simulink model "HeatExchanger"  (Simulink 8.3)
settings: Solver=ode4  StartTime=0.0  StopTime=10  FixedStep=delta_t  RelTol=1e-3
values from neighbouring files (symbols this model uses):
  delta_t = 1 / sensor_sampling_rate    (= 0.001)    [HeatExchanger_ps.m]    (also in steady_data_76rssi_30_1.mat = 0.1; steady_data_76rssi_40.mat = 0.1; steady_data_76rssi_iter.mat = 0.1; steady_data_76rssi_iter_reduce.mat = 0.1)
libraries: powerlib_meascontrol x3, simulink x1
settings Model: Creator=Rhine  LastModifiedBy=wangwenchen
settings OptimizationCC: ExpressionDepthLimit=2147483647
settings DebuggingCC: FcnCallInpInsideContextMsg=UseLocalSettings

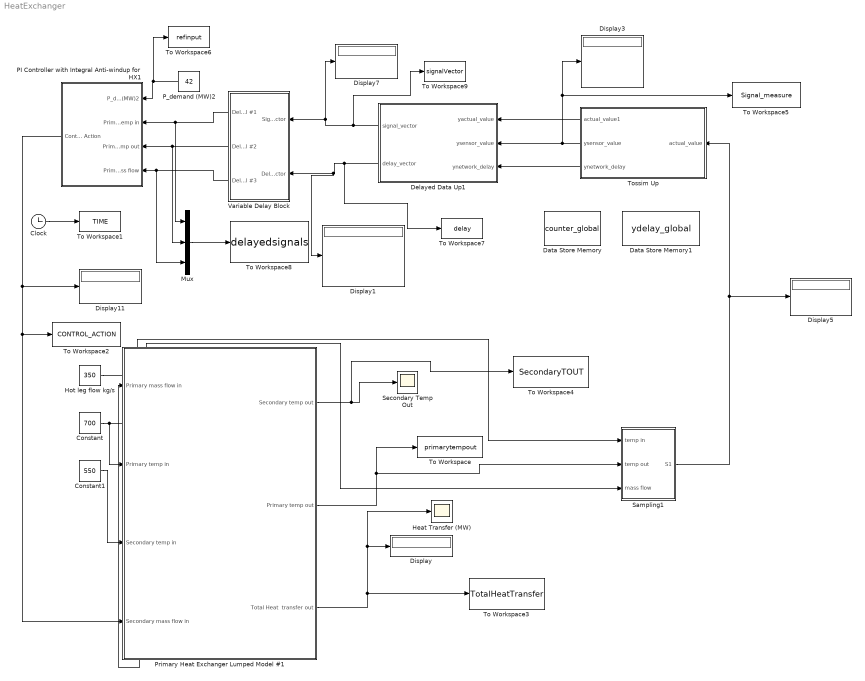
== system HeatExchanger ==
  Clock : Clock
  Constant : Constant  Value=700
  Constant1 : Constant  Value=550
  Data Store Memory : DataStoreMemory  DataStoreName=counter_global  ReadBeforeWriteMsg=warning  WriteAfterWriteMsg=warning  WriteAfterReadMsg=warning  OutDataTypeStr=int32
  Data Store Memory1 : DataStoreMemory  DataStoreName=ydelay_global  ReadBeforeWriteMsg=warning  WriteAfterWriteMsg=warning  WriteAfterReadMsg=warning  InitialValue=ones(10,1)  OutDataTypeStr=int32
  Delayed Data Up1 : MATLAB Function  TreatAsAtomicUnit=on  SystemSampleTime=0.1
  Display{,1,3,5,7,11} (6 alike) : Display
  Heat Transfer (MW) : Scope
      settings: TimeRange=30  YMin=23.3769  YMax=25.8377  SaveName=ScopeData3
  Hot leg flow kg/s : Constant  Value=350
  Mux : Mux  Inputs=3
  PI Controller with Integral Anti-windup for HX1 : Subsystem
  P_demand (MW)2 : Constant  Value=42
  Primary Heat Exchanger Lumped Model #1 : Subsystem
  Sampling1 : Subsystem
  Secondary Temp Out : Scope
      settings: YMin=639  YMax=640.4
  To Workspace : ToWorkspace  VariableName=primarytempout  SaveFormat=Timeseries  SampleTime=-1
  To Workspace1 : ToWorkspace  VariableName=TIME  SampleTime=-1
  To Workspace2 : ToWorkspace  VariableName=CONTROL_ACTION  SaveFormat=Timeseries  SampleTime=-1
  To Workspace3 : ToWorkspace  VariableName=TotalHeatTransfer  SaveFormat=Timeseries  SampleTime=-1
  To Workspace4 : ToWorkspace  VariableName=SecondaryTOUT  SaveFormat=Timeseries  SampleTime=-1
  To Workspace5 : ToWorkspace  VariableName=Signal_measure  SampleTime=-1
  To Workspace6 : ToWorkspace  VariableName=refinput  SaveFormat=Timeseries  SampleTime=-1
  To Workspace7 : ToWorkspace  VariableName=delay  SaveFormat=Timeseries  SampleTime=-1
  To Workspace8 : ToWorkspace  VariableName=delayedsignals  SaveFormat=Timeseries  SampleTime=-1
  To Workspace9 : ToWorkspace  VariableName=signalVector  SaveFormat=Timeseries  SampleTime=-1
  Tossim Up : MATLAB Function  TreatAsAtomicUnit=on  SystemSampleTime=0.1
  Variable Delay Block : Subsystem
  wires:
  Clock/1 -> To Workspace1/1
  Tossim Up/1(actual_value1) -> Delayed Data Up1/1(yactual_value)
  Sampling1/1(S1) -> Tossim Up/1(actual_value), Display5/1
  P_demand (MW)2/1 -> To Workspace6/1, PI Controller with Integral Anti-windup for HX1/1(P_demand (MW)2)
  Hot leg flow kg/s/1 -> Sampling1/3(mass flow), Primary Heat Exchanger Lumped Model #1/1(Primary mass flow in)
  Constant/1 -> Sampling1/1(temp in), Primary Heat Exchanger Lumped Model #1/2(Primary temp in)
  Constant1/1 -> Primary Heat Exchanger Lumped Model #1/3(Secondary temp in)
  Primary Heat Exchanger Lumped Model #1/2(Primary temp out) -> To Workspace/1, Sampling1/2(temp out)
  Primary Heat Exchanger Lumped Model #1/1(Secondary temp out) -> To Workspace4/1, Secondary Temp Out/1
  Variable Delay Block/1(Delayed signal #1) -> Mux/1, PI Controller with Integral Anti-windup for HX1/2(Primary temp in)
  Variable Delay Block/2(Delayed signal #2) -> PI Controller with Integral Anti-windup for HX1/3(Primary temp out), Mux/2
  Variable Delay Block/3(Delayed signal #3) -> Mux/3, PI Controller with Integral Anti-windup for HX1/4(Primary mass flow)
  PI Controller with Integral Anti-windup for HX1/1(Control Action) -> Display11/1, Primary Heat Exchanger Lumped Model #1/4(Secondary mass flow in), To Workspace2/1
  Primary Heat Exchanger Lumped Model #1/3("Total Heat  transfer out ") -> Heat Transfer (MW)/1, Display/1, To Workspace3/1
  Delayed Data Up1/1(signal_vector) -> To Workspace9/1, Display7/1, Variable Delay Block/1(Signal vector)
  Tossim Up/2(ysensor_value) -> Display3/1, To Workspace5/1, Delayed Data Up1/2(ysensor_value)
  Tossim Up/3(ynetwork_delay) -> Delayed Data Up1/3(ynetwork_delay)
  Delayed Data Up1/2(delay_vector) -> To Workspace7/1, Display1/1, Variable Delay Block/2(Delay vector)
  Mux/1 -> To Workspace8/1

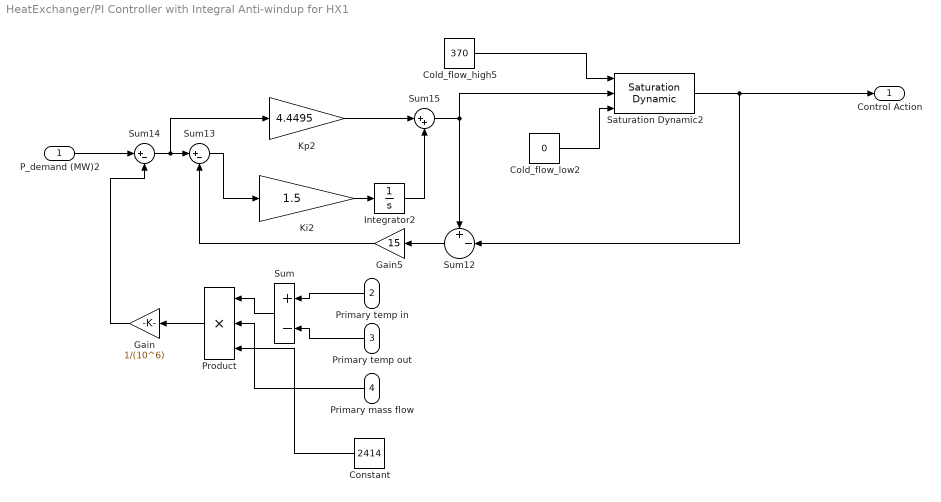
== system HeatExchanger/PI Controller with Integral Anti-windup for HX1 ==
  P_demand (MW)2 : Inport
  Primary temp in : Inport  Port=2
  Primary temp out : Inport  Port=3
  Primary mass flow : Inport  Port=4
  Cold_flow_high5 : Constant  Value=370
  Cold_flow_low2 : Constant  Value=0
  Constant : Constant  Value=2414
  Gain : Gain  Gain=1/(10^6)
  Gain5 : Gain  Gain=15
  Integrator2 : Integrator  InitialCondition=250
  Ki2 : Gain  Gain=1.5
  Kp2 : Gain  Gain=4.4495
  Product : Product  Inputs=3
  Saturation Dynamic2 : simulink/Discontinuities/Saturation Dynamic  OutMin=[]  OutMax=[]  OutDataTypeStr=Inherit: Same as second input  OutDataType=fixdt(1, 16)  OutScaling=2^-10  DoSatur=off
  Sum : Sum  Inputs=+-
  Sum12 : Sum  Inputs=+-|
  Sum13 : Sum  Inputs=|+-
  Sum14 : Sum  Inputs=|+-
  Sum15 : Sum  Inputs=|++
  Control Action : Outport
  wires:
  Product/1 -> Gain/1
  Cold_flow_low2/1 -> Saturation Dynamic2/3
  Cold_flow_high5/1 -> Saturation Dynamic2/1
  Sum14/1 -> Kp2/1, Sum13/1
  P_demand (MW)2/1 -> Sum14/1
  Sum12/1 -> Gain5/1
  Integrator2/1 -> Sum15/2
  Gain5/1 -> Sum13/2
  Sum13/1 -> Ki2/1
  Ki2/1 -> Integrator2/1
  Kp2/1 -> Sum15/1
  Saturation Dynamic2/1 -> Control Action/1, Sum12/2
  Sum15/1 -> Sum12/1, Saturation Dynamic2/2
  Primary temp in/1 -> Sum/1
  Primary temp out/1 -> Sum/2
  Sum/1 -> Product/1
  Primary mass flow/1 -> Product/2
  Constant/1 -> Product/3
  Gain/1 -> Sum14/2

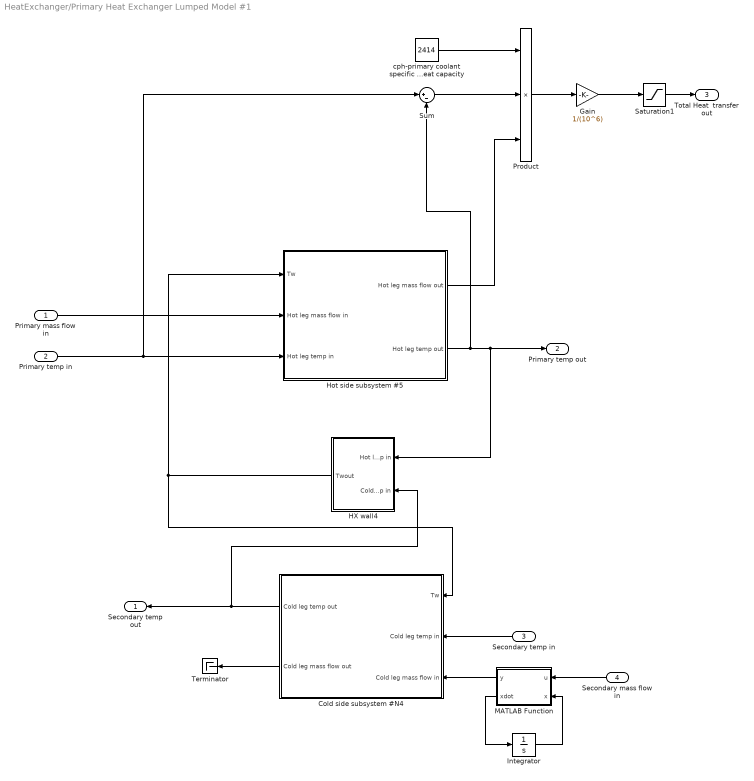
== system HeatExchanger/Primary Heat Exchanger Lumped Model #1 ==
  Primary mass flow in : Inport
  Primary temp in : Inport  Port=2
  Secondary temp in : Inport  Port=3
  Secondary mass flow in : Inport  Port=4
  Cold side subsystem #N4 : Subsystem
  Gain : Gain  Gain=1/(10^6)
  HX wall4 : Subsystem
  Hot side subsystem #5 : Subsystem
  Integrator : Integrator  InitialCondition=250
  MATLAB Function : MATLAB Function  TreatAsAtomicUnit=on
  Product : Product  Inputs=3
  Saturation1 : Saturate  UpperLimit=inf  LowerLimit=0
  Sum : Sum  Inputs=|+-
  Terminator : Terminator
  cph-primary coolant specific heat capacity : Constant  Value=2414
  Secondary temp out : Outport
  Primary temp out : Outport  Port=2
  "Total Heat  transfer out " : Outport  Port=3
  wires:
  Cold side subsystem #N4/1(Cold leg temp out) -> Secondary temp out/1, HX wall4/2(Cold leg temp in)
  Cold side subsystem #N4/2(Cold leg mass flow out) -> Terminator/1
  Primary mass flow in/1 -> Hot side subsystem #5/2(Hot leg mass flow in)
  Primary temp in/1 -> Hot side subsystem #5/3(Hot leg temp in), Sum/1
  Secondary mass flow in/1 -> MATLAB Function/1(u)
  Secondary temp in/1 -> Cold side subsystem #N4/2(Cold leg temp in)
  HX wall4/1(Twout) -> Cold side subsystem #N4/1(Tw), Hot side subsystem #5/1(Tw)
  Hot side subsystem #5/1(Hot leg mass flow out) -> Product/3
  Hot side subsystem #5/2(Hot leg temp out) -> HX wall4/1(Hot leg temp in), Primary temp out/1, Sum/2
  cph-primary coolant specific heat capacity/1 -> Product/1
  Sum/1 -> Product/2
  Product/1 -> Gain/1
  Gain/1 -> Saturation1/1
  MATLAB Function/1(y) -> Cold side subsystem #N4/3(Cold leg mass flow in)
  Saturation1/1 -> "Total Heat  transfer out "/1
  MATLAB Function/2(xdot) -> Integrator/1
  Integrator/1 -> MATLAB Function/2(x)

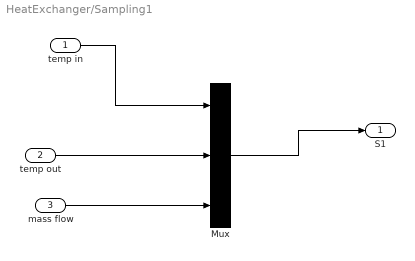
== system HeatExchanger/Sampling1 ==
  temp in : Inport
  temp out : Inport  Port=2
  mass flow : Inport  Port=3
  Mux : Mux  Inputs=3
  S1 : Outport
  wires:
  temp in/1 -> Mux/1
  temp out/1 -> Mux/2
  mass flow/1 -> Mux/3
  Mux/1 -> S1/1

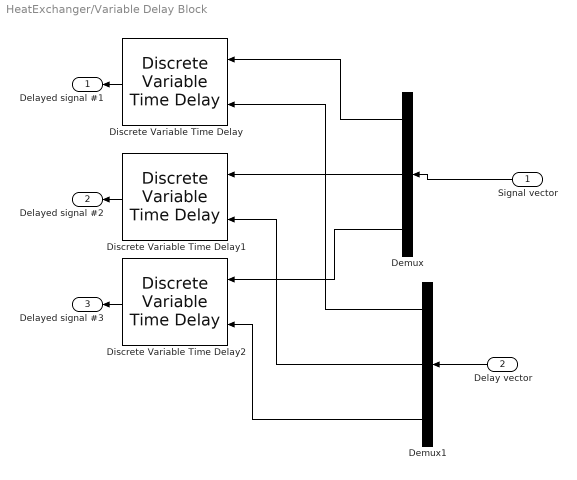
== system HeatExchanger/Variable Delay Block ==
  Signal vector : Inport
  Delay vector : Inport  Port=2
  Demux : Demux  Outputs=3
  Demux1 : Demux  Outputs=3
  Discrete Variable Time Delay : powerlib_meascontrol/Additional Components/Discrete Variable Time Delay  MaxDelay=2  InitialValue=700  Ts=delta_t  DFT=on
  Discrete Variable Time Delay1 : powerlib_meascontrol/Additional Components/Discrete Variable Time Delay  MaxDelay=2  InitialValue=650.29  Ts=delta_t  DFT=on
  Discrete Variable Time Delay2 : powerlib_meascontrol/Additional Components/Discrete Variable Time Delay  MaxDelay=2  InitialValue=350  Ts=delta_t  DFT=on
  Delayed signal #1 : Outport
  Delayed signal #2 : Outport  Port=2
  Delayed signal #3 : Outport  Port=3
  wires:
  Discrete Variable Time Delay1/1 -> Delayed signal #2/1
  Demux1/3 -> Discrete Variable Time Delay2/2
  Demux1/2 -> Discrete Variable Time Delay1/2
  Discrete Variable Time Delay2/1 -> Delayed signal #3/1
  Demux/3 -> Discrete Variable Time Delay2/1
  Demux/1 -> Discrete Variable Time Delay/1
  Demux1/1 -> Discrete Variable Time Delay/2
  Discrete Variable Time Delay/1 -> Delayed signal #1/1
  Signal vector/1 -> Demux/1
  Demux/2 -> Discrete Variable Time Delay1/1
  Delay vector/1 -> Demux1/1

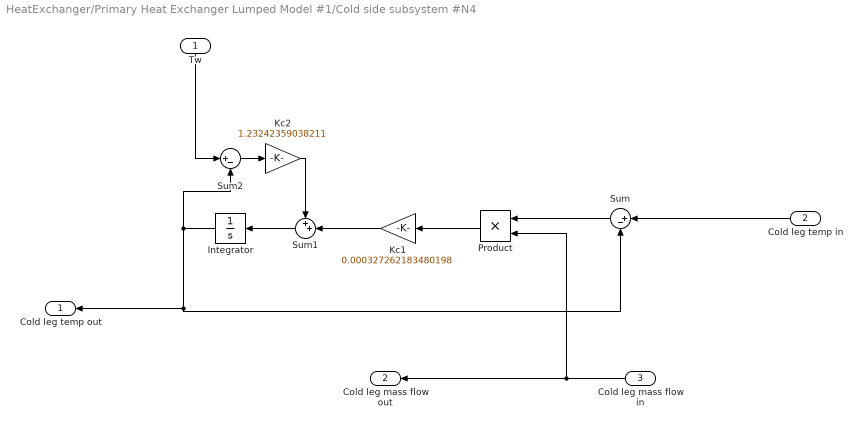
== system HeatExchanger/Primary Heat Exchanger Lumped Model #1/Cold side subsystem #N4 ==
  Tw : Inport
  Cold leg temp in : Inport  Port=2
  Cold leg mass flow in : Inport  Port=3
  Integrator : Integrator  InitialCondition=638.4
  Kc1 : Gain  Gain=0.000327262183480198
  Kc2 : Gain  Gain=1.23242359038211
  Product : Product
  Sum : Sum  Inputs=|+-
  Sum1 : Sum  Inputs=++|
  Sum2 : Sum  Inputs=|+-
  Cold leg temp out : Outport
  Cold leg mass flow out : Outport  Port=2
  wires:
  Cold leg temp in/1 -> Sum/1
  Integrator/1 -> Sum/2, Cold leg temp out/1, Sum2/2
  Sum2/1 -> Kc2/1
  Sum/1 -> Product/1
  Kc2/1 -> Sum1/1
  Sum1/1 -> Integrator/1
  Cold leg mass flow in/1 -> Cold leg mass flow out/1, Product/2
  Product/1 -> Kc1/1
  Kc1/1 -> Sum1/2
  Tw/1 -> Sum2/1

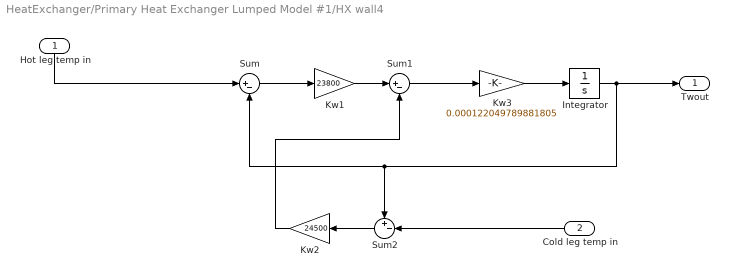
== system HeatExchanger/Primary Heat Exchanger Lumped Model #1/HX wall4 ==
  Hot leg temp in : Inport
  Cold leg temp in : Inport  Port=2
  Integrator : Integrator  InitialCondition=644.3
  Kw1 : Gain  Gain=23800
  Kw2 : Gain  Gain=24500
  Kw3 : Gain  Gain=0.000122049789881805
  Sum : Sum  Inputs=|+-
  Sum1 : Sum  Inputs=|+-
  Sum2 : Sum  Inputs=+-|
  Twout : Outport
  wires:
  Sum2/1 -> Kw2/1
  Hot leg temp in/1 -> Sum/1
  Sum1/1 -> Kw3/1
  Cold leg temp in/1 -> Sum2/2
  Sum/1 -> Kw1/1
  Kw1/1 -> Sum1/1
  Kw3/1 -> Integrator/1
  Integrator/1 -> Twout/1, Sum2/1, Sum/2
  Kw2/1 -> Sum1/2

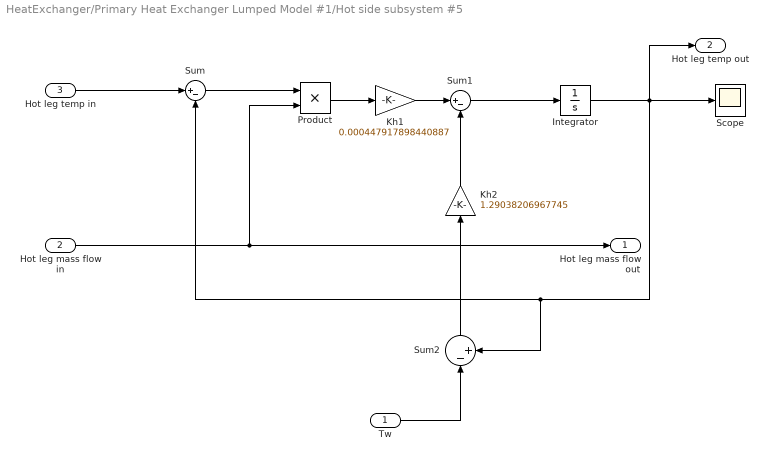
== system HeatExchanger/Primary Heat Exchanger Lumped Model #1/Hot side subsystem #5 ==
  Tw : Inport
  Hot leg mass flow in : Inport  Port=2
  Hot leg temp in : Inport  Port=3
  Integrator : Integrator  InitialCondition=650.29
  Kh1 : Gain  Gain=0.000447917898440887
  Kh2 : Gain  Gain=1.29038206967745
  Product : Product
  Scope : Scope
  Sum : Sum  Inputs=|+-
  Sum1 : Sum  Inputs=|+-
  Sum2 : Sum  Inputs=|-+
  Hot leg mass flow out : Outport
  Hot leg temp out : Outport  Port=2
  wires:
  Product/1 -> Kh1/1
  Kh1/1 -> Sum1/1
  Sum1/1 -> Integrator/1
  Sum2/1 -> Kh2/1
  Kh2/1 -> Sum1/2
  Tw/1 -> Sum2/1
  Hot leg temp in/1 -> Sum/1
  Hot leg mass flow in/1 -> Hot leg mass flow out/1, Product/2
  Sum/1 -> Product/1
  Integrator/1 -> Hot leg temp out/1, Scope/1, Sum2/2, Sum/2

== matlab function Tossim Up ==
  data: actual_value1 output double; actual_value input double; ysensor_value output double; ydelay_global data_store_memory double; counter_global data_store_memory double; ynetwork_delay output double
function [actual_value1, ysensor_value, ynetwork_delay]  = Tossim_block(actual_value)

% Inputs:
% ymea: measurement from structure

% Outputs:
% ymea1: measurement output
% ydelay: delay traces

persistent sensor_value % delay trace
persistent i  
% count
global ydelay_global
global counter_global

% allow these matlab functions to be used in Embedded Matlab block
eml.extrinsic('python');
eml.extrinsic('num2str');
eml.extrinsic('str2num');
eml.extrinsic('delay_summary');
eml.extrinsic('disp');
eml.extrinsic('ps_aggregation');
eml.extrinsic('for');
eml.extrinsic('end');

if isempty(i)
    i = 0;
end

%sen_num=structure.sen_num;

ysensor_value = [0 0 0]'; 
ynetwork_delay = [0 0 0]';



call_count = 56; % number of slots + 1 (i.e., number of client calls made + 1) per TDMA schedule, +1 to have full 53 slots after %

[resultz] = ps_aggregation(call_count);


%end_to_end_delivery_result_aggregated = sum(resultz);
end_to_end_delivery_result_aggregated=resultz;

[sensor_value_tmp] = value_summary(end_to_end_delivery_result_aggregated);
ysensor_value = sensor_value_tmp';

[network_delay_tmp] = network_delay_summary(end_to_end_delivery_result_aggregated);
%disp(network_delay)
ynetwork_delay=network_delay_tmp';

disp('sensor_value')
disp(ysensor_value')
%disp('network delay')
%disp(ynetwork_delay')
disp('------------i------------')
disp(i)

%last_emergency_instance = ymea';
sensor_value = ysensor_value;
i = i + 1;

actual_value1 = [0 0 0]'; %3 sensors
actual_value1 = actual_value;


for h_yg = 1:3
    ydelay_global(h_yg, 1) = ysensor_value(h_yg, 1);
end

disp('Plant 1, TOSSIM Uplink Block, is called');
counter_global = counter_global + 1;

== matlab function Primary Heat Exchanger Lumped Model #1/MATLAB Function ==
  data: u input double; y output double; x input double; xdot output double
function [y,xdot] = pump(u,x)
%#codegen

if u<0
    u=0;
else
end

xdot = -0.1*x + 0.1*u;

y = x;

== matlab function Delayed Data Up1 ==
  data: yactual_value input double; ysensor_value input double; ynetwork_delay input double; signal_vector output double; structure parameter double; delay_vector output double
function [signal_vector, delay_vector] = delay_block(yactual_value,ysensor_value, ynetwork_delay, structure)

% Inputs: 
% yactual_value: measurements output
% yactual_value: sensor value traces
% ynetwork_delay: delay traces
% structure: other necessary information 

% Outputs:
% signal_vector: sensor measurments
% delay_vector: delay value
persistent  i yin_d delay_v
persistent yin sensor_value num ynd_tmp
persistent last_senReading last_senDelay
%global yin_all ynd_all

eml.extrinsic('disp');
eml.extrinsic('putvar');



% sennum=5;  %number of the sensors
%step_count = 1000; %step_count
%sen_num=9;
% initialize parameters
if isempty(yin)
    i = structure.i;
    yin = structure.yin;    
    ynd_tmp= structure.ynd_tmp;

    yin_d = structure.yin_d; 
    delay_v = structure.delay_v;
    
    last_senReading = zeros(1,9);
    last_senDelay = zeros(1,9);
    
    %yin_all = structure.yin_all; %zeros (step count, sensor number)
    %ynd_all=structure.ynd_all;
    
    %yin_all = zeros(step_count+1,9); %zeros (step count, sensor number)
    %ynd_all=zeros(step_count+1,9);
    
    sensor_value = zeros(1,3);         %initialized
    sensor_value = ysensor_value';
    num = 0;
end

%yin_all = zeros(step_count+1,9); %zeros (step count, sensor number)
%ynd_all=zeros(step_count+1,9);

sensor_reading=[0 0 0];
sensor_delay=[0 0 0];
num = num+1;   

%get delay information 
% delay=zeros(1,10+1); 
sensor_value=ysensor_value';
    

%get value from "yactual_value" input
if num == 1
    for kk = 1:3
        last_senReading(kk) = yactual_value(kk); %offset=5
        last_senDelay(kk) = ynetwork_delay(kk);
    end 
end
%generate output value according to delay    
for j=1:3
    if sensor_value(1,j)~=88
        last_senReading(j) = yactual_value(j);
        last_senDelay(j) = ynetwork_delay(j);
        yin(j) = last_senReading(j);  %packet receive
        ynd_tmp(j)=last_senDelay(j);
        
    else
        if num>1 
             yin(j)=last_senReading(j); %if lost, set it to previous value
             last_senReading(j)=last_senReading(j);
             ynd_tmp(j)=last_senDelay(j)+0.1;
             last_senDelay(j)=last_senDelay(j)+0.1;
        end        
    end
end

avg_delay=0.0;

for kk = 1:3
    %sensor_reading(kk)= yin_all(num,kk); %offset=5
    %sensor_delay(kk) = ynd_all(num,kk);
    avg_delay =last_senDelay(kk)+avg_delay;

end

avg_delay = avg_delay/3.0;
fileID = fopen('sensor_data.txt','a');
fprintf(fileID, '%f\n', avg_delay);
fclose(fileID);

%putvar(yin_all, ynd_all);

%structure.yin_all=yin_all;
%structure.ynd_all=ynd_all;

yin_d = yin';
delay_v = ynd_tmp';
%delay_v = ynd_tmp'/3;
%delay_v = [0,0,0]';

signal_vector = yin_d;

delay_vector = delay_v;

disp('converted sensor_value')
disp(signal_vector')
disp('converted network delay')
disp(delay_vector')
disp('---------------num-------------')
disp(num)

% disp('plant2');

% yout_delay'
i = i+1;
